simulink model "RotorModel"  (R2021a)
settings: Solver=VariableStepAuto  StartTime=0.0  StopTime=0.5  RelTol=1e-3
model workspace (MAT data in the model file):
  D = 0.711
  DragCoeff = 4e-05
  J = 0.003408
  Ke = 0.0796
  Kt = 0.079
  La = 4.55e-05
  LiftCoeff = 0.0026
  Ra = 0.06
  Rho = 1.2256
  kf = 0.03408
settings Model: Creator=js20164  LastModifiedBy=james
settings SolverCC: AlgebraicLoopSolver=TrustRegion
settings DebuggingCC: SFMachineParentedDataDiag=warning

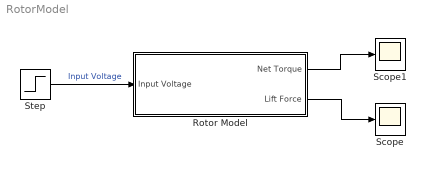
== system RotorModel ==
  Rotor Model : Subsystem
  Scope : Scope
  Scope1 : Scope
  Step : Step  Time=0.1  SampleTime=0
  wires:
  Step/1 -> Rotor Model/1(Input Voltage)  "Input Voltage"
  Rotor Model/1(Net Torque) -> Scope1/1
  Rotor Model/2(Lift Force) -> Scope/1

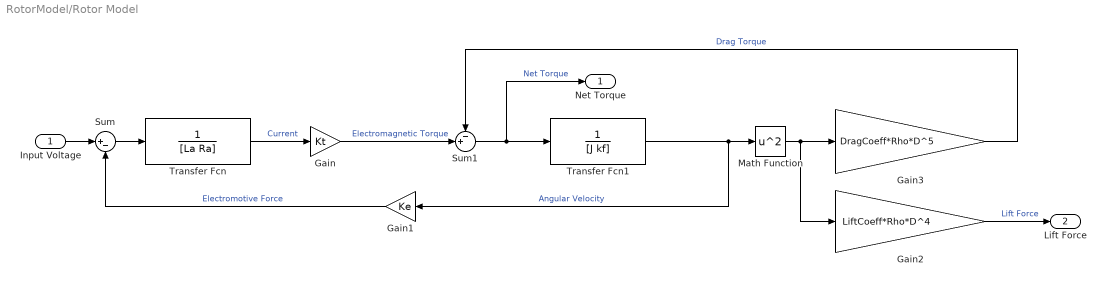
== system RotorModel/Rotor Model ==
  Input Voltage : Inport
  Gain : Gain  Gain=Kt
  Gain1 : Gain  Gain=Ke
  Gain2 : Gain  Gain=LiftCoeff*Rho*D^4
  Gain3 : Gain  Gain=DragCoeff*Rho*D^5
  Math Function : Math  Operator=square  SaturateOnIntegerOverflow=on
  Sum : Sum  Inputs=|+-
  Sum1 : Sum  Inputs=-+|
  Transfer Fcn : TransferFcn  Denominator=[La Ra]
  Transfer Fcn1 : TransferFcn  Denominator=[J kf]
  Net Torque : Outport
  Lift Force : Outport  Port=2
  wires:
  Gain1/1 -> Sum/2  "Electromotive Force"
  Input Voltage/1 -> Sum/1
  Sum/1 -> Transfer Fcn/1
  Gain2/1 -> Lift Force/1  "Lift Force"
  Gain3/1 -> Sum1/1  "Drag Torque"
  Gain/1 -> Sum1/2  "Electromagnetic Torque"
  Sum1/1 -> Net Torque/1, Transfer Fcn1/1  "Net Torque"
  Transfer Fcn1/1 -> Gain1/1, Math Function/1  "Angular Velocity"
  Math Function/1 -> Gain3/1, Gain2/1
  Transfer Fcn/1 -> Gain/1  "Current"
